simulink model "lab3"  (R2025b)
settings: Solver=ode1  StartTime=0.0  StopTime=100.0  FixedStep=0.1  RelTol=1e-3
settings Model: Creator=mizula  LastModifiedBy=mizula

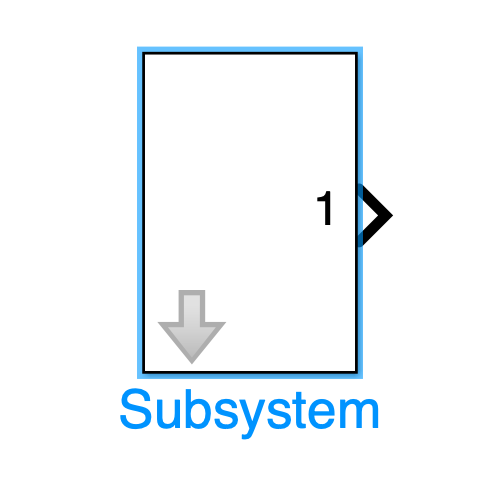
[thumbnail: Simulink's stored preview of the top-level diagram]
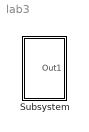
== system lab3 ==
  Subsystem : Subsystem  mask{y=180, k=1, l=3, m=10, g=10}

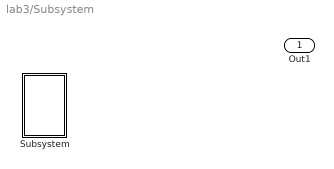
== system lab3/Subsystem ==
  Subsystem : Subsystem
  Out1 : Outport
  wires:
  ? -> Out1/1

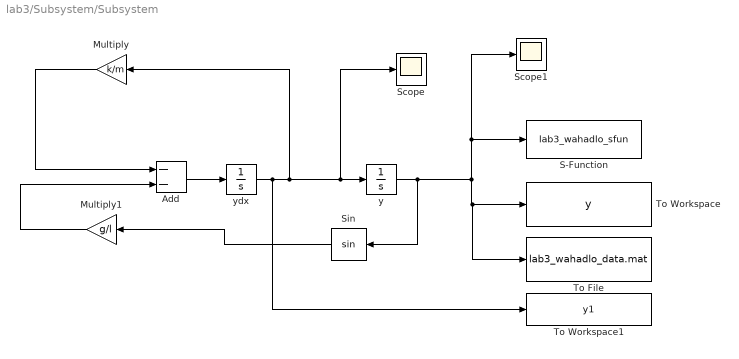
== system lab3/Subsystem/Subsystem ==
  Add : Sum  Inputs=--
  Multiply : Gain  Gain=k/m
  Multiply1 : Gain  Gain=g/l
  S-Function : S-Function  FunctionName=lab3_wahadlo_sfun  Parameters=l,m,y  SFunctionDeploymentMode=off  EnableBusSupport=off
  Scope : Scope
      settings: ActiveDisplayYMinimum=-60.027369909356295  ActiveDisplayYMaximum=26.944607586906844
  Scope1 : Scope
      settings: ActiveDisplayYMinimum=-170.51394580243107  ActiveDisplayYMaximum=22.016032753128652
  Sin : Trigonometry
  To File : ToFile  Filename=lab3_wahadlo_data.mat  SaveFormat=Timeseries
  To Workspace : ToWorkspace  VariableName=y  SaveFormat=Timeseries  SampleTime=-1
  To Workspace1 : ToWorkspace  VariableName=y1  SaveFormat=Timeseries  SampleTime=-1
  y : Integrator  InitialCondition=y*pi/180
  ydx : Integrator
  wires:
  Multiply1/1 -> Add/2
  ydx/1 -> To Workspace1/1, Multiply/1, Scope/1, y/1
  Multiply/1 -> Add/1
  Add/1 -> ydx/1
  y/1 -> Sin/1, To File/1, To Workspace/1, Scope1/1, S-Function/1
  Sin/1 -> Multiply1/1
